simulink model "c00003M_harness"  (R2018a)
settings: Solver=FixedStepAuto  StartTime=0.0  StopTime=300  FixedStep=0.1  RelTol=1e-3
undefined symbols (not defined in the file): A1, hmax, PriorityTank, R1, R2, sigbuilder_block
(part 8 of 44)

== system c00003M_harness/M006/Tank1 ==
  CT1 : Inport
  F1 : Inport  Port=2
  E1 : Inport  Port=3
  MR1 : Inport  Port=4
  T1 : Inport  Port=5
  EB1 : Inport  Port=6
  LL2 : Inport  Port=7
  Control : Subsystem
  Logical Operator : Logic  AllPortsSameDT=off  OutDataTypeStr=boolean
  MasterTankControl : Subsystem
  Memory : Memory
  Memory1 : Memory
  TankModel : Subsystem
  LL1 : Outport
  wires:
  TankModel/1(LiquidLevel) -> Memory/1, LL1/1
  Control/1(LiquidIn) -> Logical Operator/1
  Control/2(LiquidOut) -> TankModel/2(LiquidOut)
  Memory/1 -> Control/7(LiquidLevel), MasterTankControl/1(LiquidTank1)
  MR1/1 -> Control/3(ManualReference)
  CT1/1 -> Control/2(StartMaintenance), Control/1(ControlType)
  F1/1 -> Control/4(Fill)
  E1/1 -> Control/5(Empty)
  Memory1/1 -> MasterTankControl/2(LiquidTank2)
  EB1/1 -> Control/6(EmergencyButton)
  MasterTankControl/1(AllowTheTankFilling) -> Logical Operator/2
  Logical Operator/1 -> TankModel/1(LiquidIn)
  LL2/1 -> Memory1/1

== system c00003M_harness/M006/Tank2 ==
  CT2 : Inport
  F2 : Inport  Port=2
  E2 : Inport  Port=3
  MR2 : Inport  Port=4
  T2 : Inport  Port=5
  EB2 : Inport  Port=6
  LL1 : Inport  Port=7
  Control : Subsystem
  Logical Operator : Logic  AllPortsSameDT=off  OutDataTypeStr=boolean
  MasterTankControl : Subsystem
  Memory : Memory
  Memory1 : Memory
  TankModel : Subsystem
  LL2 : Outport
  wires:
  TankModel/1(LiquidLevel) -> Memory/1, LL2/1
  Control/1(LiquidIn) -> Logical Operator/1
  Control/2(LiquidOut) -> TankModel/2(LiquidOut)
  Memory/1 -> Control/6(LiquidLevel), MasterTankControl/2(LiquidTank2)
  MR2/1 -> Control/2(ManualReference)
  CT2/1 -> Control/1(ControlType)
  F2/1 -> Control/3(Fill)
  E2/1 -> Control/4(Empty)
  Memory1/1 -> MasterTankControl/1(LiquidTank1)
  EB2/1 -> Control/5(EmergencyButton)
  MasterTankControl/1(AllowTheTankFilling) -> Logical Operator/2
  Logical Operator/1 -> TankModel/1(LiquidIn)
  LL1/1 -> Memory1/1

== system c00003M_harness/M007/Tank1 ==
  CT1 : Inport
  F1 : Inport  Port=2
  E1 : Inport  Port=3
  MR1 : Inport  Port=4
  T1 : Inport  Port=5
  EB1 : Inport  Port=6
  LL2 : Inport  Port=7
  Control : Subsystem
  Logical Operator : Logic  AllPortsSameDT=off  OutDataTypeStr=boolean
  MasterTankControl : Subsystem
  Memory : Memory
  Memory1 : Memory
  TankModel : Subsystem
  LL1 : Outport
  wires:
  TankModel/1(LiquidLevel) -> Memory/1, LL1/1
  Control/1(LiquidIn) -> Logical Operator/1
  Control/2(LiquidOut) -> TankModel/2(LiquidOut)
  Memory/1 -> Control/7(LiquidLevel), MasterTankControl/1(LiquidTank1)
  MR1/1 -> Control/3(ManualReference)
  CT1/1 -> Control/2(StartMaintenance), Control/1(ControlType)
  F1/1 -> Control/4(Fill)
  E1/1 -> Control/5(Empty)
  Memory1/1 -> MasterTankControl/2(LiquidTank2)
  EB1/1 -> Control/6(EmergencyButton)
  MasterTankControl/1(AllowTheTankFilling) -> Logical Operator/2
  Logical Operator/1 -> TankModel/1(LiquidIn)
  LL2/1 -> Memory1/1

== system c00003M_harness/M007/Tank2 ==
  CT2 : Inport
  F2 : Inport  Port=2
  E2 : Inport  Port=3
  MR2 : Inport  Port=4
  T2 : Inport  Port=5
  EB2 : Inport  Port=6
  LL1 : Inport  Port=7
  Control : Subsystem
  Logical Operator : Logic  AllPortsSameDT=off  OutDataTypeStr=boolean
  MasterTankControl : Subsystem
  Memory : Memory
  Memory1 : Memory
  TankModel : Subsystem
  LL2 : Outport
  wires:
  TankModel/1(LiquidLevel) -> Memory/1, LL2/1
  Control/1(LiquidIn) -> Logical Operator/1
  Control/2(LiquidOut) -> TankModel/2(LiquidOut)
  Memory/1 -> Control/6(LiquidLevel), MasterTankControl/2(LiquidTank2)
  MR2/1 -> Control/2(ManualReference)
  CT2/1 -> Control/1(ControlType)
  F2/1 -> Control/3(Fill)
  E2/1 -> Control/4(Empty)
  Memory1/1 -> MasterTankControl/1(LiquidTank1)
  EB2/1 -> Control/5(EmergencyButton)
  MasterTankControl/1(AllowTheTankFilling) -> Logical Operator/2
  Logical Operator/1 -> TankModel/1(LiquidIn)
  LL1/1 -> Memory1/1

== system c00003M_harness/M008/Tank1 ==
  CT1 : Inport
  F1 : Inport  Port=2
  E1 : Inport  Port=3
  MR1 : Inport  Port=4
  T1 : Inport  Port=5
  EB1 : Inport  Port=6
  LL2 : Inport  Port=7
  Control : Subsystem
  Logical Operator : Logic  AllPortsSameDT=off  OutDataTypeStr=boolean
  MasterTankControl : Subsystem
  Memory : Memory
  Memory1 : Memory
  TankModel : Subsystem
  LL1 : Outport
  wires:
  TankModel/1(LiquidLevel) -> Memory/1, LL1/1
  Control/1(LiquidIn) -> Logical Operator/1
  Control/2(LiquidOut) -> TankModel/2(LiquidOut)
  Memory/1 -> Control/7(LiquidLevel), MasterTankControl/1(LiquidTank1)
  MR1/1 -> Control/3(ManualReference)
  CT1/1 -> Control/2(StartMaintenance), Control/1(ControlType)
  F1/1 -> Control/4(Fill)
  E1/1 -> Control/5(Empty)
  Memory1/1 -> MasterTankControl/2(LiquidTank2)
  EB1/1 -> Control/6(EmergencyButton)
  MasterTankControl/1(AllowTheTankFilling) -> Logical Operator/2
  Logical Operator/1 -> TankModel/1(LiquidIn)
  LL2/1 -> Memory1/1

== system c00003M_harness/M008/Tank2 ==
  CT2 : Inport
  F2 : Inport  Port=2
  E2 : Inport  Port=3
  MR2 : Inport  Port=4
  T2 : Inport  Port=5
  EB2 : Inport  Port=6
  LL1 : Inport  Port=7
  Control : Subsystem
  Logical Operator : Logic  AllPortsSameDT=off  OutDataTypeStr=boolean
  MasterTankControl : Subsystem
  Memory : Memory
  Memory1 : Memory
  TankModel : Subsystem
  LL2 : Outport
  wires:
  TankModel/1(LiquidLevel) -> Memory/1, LL2/1
  Control/1(LiquidIn) -> Logical Operator/1
  Control/2(LiquidOut) -> TankModel/2(LiquidOut)
  Memory/1 -> Control/6(LiquidLevel), MasterTankControl/2(LiquidTank2)
  MR2/1 -> Control/2(ManualReference)
  CT2/1 -> Control/1(ControlType)
  F2/1 -> Control/3(Fill)
  E2/1 -> Control/4(Empty)
  Memory1/1 -> MasterTankControl/1(LiquidTank1)
  EB2/1 -> Control/5(EmergencyButton)
  MasterTankControl/1(AllowTheTankFilling) -> Logical Operator/2
  Logical Operator/1 -> TankModel/1(LiquidIn)
  LL1/1 -> Memory1/1

== system c00003M_harness/M009/Tank1 ==
  CT1 : Inport
  F1 : Inport  Port=2
  E1 : Inport  Port=3
  MR1 : Inport  Port=4
  T1 : Inport  Port=5
  EB1 : Inport  Port=6
  LL2 : Inport  Port=7
  Control : Subsystem
  Logical Operator : Logic  AllPortsSameDT=off  OutDataTypeStr=boolean
  MasterTankControl : Subsystem
  Memory : Memory
  Memory1 : Memory
  TankModel : Subsystem
  LL1 : Outport
  wires:
  TankModel/1(LiquidLevel) -> Memory/1, LL1/1
  Control/1(LiquidIn) -> Logical Operator/1
  Control/2(LiquidOut) -> TankModel/2(LiquidOut)
  Memory/1 -> Control/7(LiquidLevel), MasterTankControl/1(LiquidTank1)
  MR1/1 -> Control/3(ManualReference)
  CT1/1 -> Control/2(StartMaintenance), Control/1(ControlType)
  F1/1 -> Control/4(Fill)
  E1/1 -> Control/5(Empty)
  Memory1/1 -> MasterTankControl/2(LiquidTank2)
  EB1/1 -> Control/6(EmergencyButton)
  MasterTankControl/1(AllowTheTankFilling) -> Logical Operator/2
  Logical Operator/1 -> TankModel/1(LiquidIn)
  LL2/1 -> Memory1/1

== system c00003M_harness/M009/Tank2 ==
  CT2 : Inport
  F2 : Inport  Port=2
  E2 : Inport  Port=3
  MR2 : Inport  Port=4
  T2 : Inport  Port=5
  EB2 : Inport  Port=6
  LL1 : Inport  Port=7
  Control : Subsystem
  Logical Operator : Logic  AllPortsSameDT=off  OutDataTypeStr=boolean
  MasterTankControl : Subsystem
  Memory : Memory
  Memory1 : Memory
  TankModel : Subsystem
  LL2 : Outport
  wires:
  TankModel/1(LiquidLevel) -> Memory/1, LL2/1
  Control/1(LiquidIn) -> Logical Operator/1
  Control/2(LiquidOut) -> TankModel/2(LiquidOut)
  Memory/1 -> Control/6(LiquidLevel), MasterTankControl/2(LiquidTank2)
  MR2/1 -> Control/2(ManualReference)
  CT2/1 -> Control/1(ControlType)
  F2/1 -> Control/3(Fill)
  E2/1 -> Control/4(Empty)
  Memory1/1 -> MasterTankControl/1(LiquidTank1)
  EB2/1 -> Control/5(EmergencyButton)
  MasterTankControl/1(AllowTheTankFilling) -> Logical Operator/2
  Logical Operator/1 -> TankModel/1(LiquidIn)
  LL1/1 -> Memory1/1

== system c00003M_harness/M010/Tank1 ==
  CT1 : Inport
  F1 : Inport  Port=2
  E1 : Inport  Port=3
  MR1 : Inport  Port=4
  T1 : Inport  Port=5
  EB1 : Inport  Port=6
  LL2 : Inport  Port=7
  Control : Subsystem
  Logical Operator : Logic  AllPortsSameDT=off  OutDataTypeStr=boolean
  MasterTankControl : Subsystem
  Memory : Memory
  Memory1 : Memory
  TankModel : Subsystem
  LL1 : Outport
  wires:
  TankModel/1(LiquidLevel) -> Memory/1, LL1/1
  Control/1(LiquidIn) -> Logical Operator/1
  Control/2(LiquidOut) -> TankModel/2(LiquidOut)
  Memory/1 -> Control/7(LiquidLevel), MasterTankControl/1(LiquidTank1)
  MR1/1 -> Control/3(ManualReference)
  CT1/1 -> Control/2(StartMaintenance), Control/1(ControlType)
  F1/1 -> Control/4(Fill)
  E1/1 -> Control/5(Empty)
  Memory1/1 -> MasterTankControl/2(LiquidTank2)
  EB1/1 -> Control/6(EmergencyButton)
  MasterTankControl/1(AllowTheTankFilling) -> Logical Operator/2
  Logical Operator/1 -> TankModel/1(LiquidIn)
  LL2/1 -> Memory1/1

== system c00003M_harness/M010/Tank2 ==
  CT2 : Inport
  F2 : Inport  Port=2
  E2 : Inport  Port=3
  MR2 : Inport  Port=4
  T2 : Inport  Port=5
  EB2 : Inport  Port=6
  LL1 : Inport  Port=7
  Control : Subsystem
  Logical Operator : Logic  AllPortsSameDT=off  OutDataTypeStr=boolean
  MasterTankControl : Subsystem
  Memory : Memory
  Memory1 : Memory
  TankModel : Subsystem
  LL2 : Outport
  wires:
  TankModel/1(LiquidLevel) -> Memory/1, LL2/1
  Control/1(LiquidIn) -> Logical Operator/1
  Control/2(LiquidOut) -> TankModel/2(LiquidOut)
  Memory/1 -> Control/6(LiquidLevel), MasterTankControl/2(LiquidTank2)
  MR2/1 -> Control/2(ManualReference)
  CT2/1 -> Control/1(ControlType)
  F2/1 -> Control/3(Fill)
  E2/1 -> Control/4(Empty)
  Memory1/1 -> MasterTankControl/1(LiquidTank1)
  EB2/1 -> Control/5(EmergencyButton)
  MasterTankControl/1(AllowTheTankFilling) -> Logical Operator/2
  Logical Operator/1 -> TankModel/1(LiquidIn)
  LL1/1 -> Memory1/1

== system c00003M_harness/M011/Tank1 ==
  CT1 : Inport
  F1 : Inport  Port=2
  E1 : Inport  Port=3
  MR1 : Inport  Port=4
  T1 : Inport  Port=5
  EB1 : Inport  Port=6
  LL2 : Inport  Port=7
  Control : Subsystem
  Logical Operator : Logic  AllPortsSameDT=off  OutDataTypeStr=boolean
  MasterTankControl : Subsystem
  Memory : Memory
  Memory1 : Memory
  TankModel : Subsystem
  LL1 : Outport
  wires:
  TankModel/1(LiquidLevel) -> Memory/1, LL1/1
  Control/1(LiquidIn) -> Logical Operator/1
  Control/2(LiquidOut) -> TankModel/2(LiquidOut)
  Memory/1 -> Control/7(LiquidLevel), MasterTankControl/1(LiquidTank1)
  MR1/1 -> Control/3(ManualReference)
  CT1/1 -> Control/2(StartMaintenance), Control/1(ControlType)
  F1/1 -> Control/4(Fill)
  E1/1 -> Control/5(Empty)
  Memory1/1 -> MasterTankControl/2(LiquidTank2)
  EB1/1 -> Control/6(EmergencyButton)
  MasterTankControl/1(AllowTheTankFilling) -> Logical Operator/2
  Logical Operator/1 -> TankModel/1(LiquidIn)
  LL2/1 -> Memory1/1

== system c00003M_harness/M011/Tank2 ==
  CT2 : Inport
  F2 : Inport  Port=2
  E2 : Inport  Port=3
  MR2 : Inport  Port=4
  T2 : Inport  Port=5
  EB2 : Inport  Port=6
  LL1 : Inport  Port=7
  Control : Subsystem
  Logical Operator : Logic  AllPortsSameDT=off  OutDataTypeStr=boolean
  MasterTankControl : Subsystem
  Memory : Memory
  Memory1 : Memory
  TankModel : Subsystem
  LL2 : Outport
  wires:
  TankModel/1(LiquidLevel) -> Memory/1, LL2/1
  Control/1(LiquidIn) -> Logical Operator/1
  Control/2(LiquidOut) -> TankModel/2(LiquidOut)
  Memory/1 -> Control/6(LiquidLevel), MasterTankControl/2(LiquidTank2)
  MR2/1 -> Control/2(ManualReference)
  CT2/1 -> Control/1(ControlType)
  F2/1 -> Control/3(Fill)
  E2/1 -> Control/4(Empty)
  Memory1/1 -> MasterTankControl/1(LiquidTank1)
  EB2/1 -> Control/5(EmergencyButton)
  MasterTankControl/1(AllowTheTankFilling) -> Logical Operator/2
  Logical Operator/1 -> TankModel/1(LiquidIn)
  LL1/1 -> Memory1/1

== system c00003M_harness/M012/Tank1 ==
  CT1 : Inport
  F1 : Inport  Port=2
  E1 : Inport  Port=3
  MR1 : Inport  Port=4
  T1 : Inport  Port=5
  EB1 : Inport  Port=6
  LL2 : Inport  Port=7
  Control : Subsystem
  Logical Operator : Logic  AllPortsSameDT=off  OutDataTypeStr=boolean
  MasterTankControl : Subsystem
  Memory : Memory
  Memory1 : Memory
  TankModel : Subsystem
  LL1 : Outport
  wires:
  TankModel/1(LiquidLevel) -> Memory/1, LL1/1
  Control/1(LiquidIn) -> Logical Operator/1
  Control/2(LiquidOut) -> TankModel/2(LiquidOut)
  Memory/1 -> Control/7(LiquidLevel), MasterTankControl/1(LiquidTank1)
  MR1/1 -> Control/3(ManualReference)
  CT1/1 -> Control/2(StartMaintenance), Control/1(ControlType)
  F1/1 -> Control/4(Fill)
  E1/1 -> Control/5(Empty)
  Memory1/1 -> MasterTankControl/2(LiquidTank2)
  EB1/1 -> Control/6(EmergencyButton)
  MasterTankControl/1(AllowTheTankFilling) -> Logical Operator/2
  Logical Operator/1 -> TankModel/1(LiquidIn)
  LL2/1 -> Memory1/1

== system c00003M_harness/M012/Tank2 ==
  CT2 : Inport
  F2 : Inport  Port=2
  E2 : Inport  Port=3
  MR2 : Inport  Port=4
  T2 : Inport  Port=5
  EB2 : Inport  Port=6
  LL1 : Inport  Port=7
  Control : Subsystem
  Logical Operator : Logic  AllPortsSameDT=off  OutDataTypeStr=boolean
  MasterTankControl : Subsystem
  Memory : Memory
  Memory1 : Memory
  TankModel : Subsystem
  LL2 : Outport
  wires:
  TankModel/1(LiquidLevel) -> Memory/1, LL2/1
  Control/1(LiquidIn) -> Logical Operator/1
  Control/2(LiquidOut) -> TankModel/2(LiquidOut)
  Memory/1 -> Control/6(LiquidLevel), MasterTankControl/2(LiquidTank2)
  MR2/1 -> Control/2(ManualReference)
  CT2/1 -> Control/1(ControlType)
  F2/1 -> Control/3(Fill)
  E2/1 -> Control/4(Empty)
  Memory1/1 -> MasterTankControl/1(LiquidTank1)
  EB2/1 -> Control/5(EmergencyButton)
  MasterTankControl/1(AllowTheTankFilling) -> Logical Operator/2
  Logical Operator/1 -> TankModel/1(LiquidIn)
  LL1/1 -> Memory1/1

== system c00003M_harness/M013/Tank1 ==
  CT1 : Inport
  F1 : Inport  Port=2
  E1 : Inport  Port=3
  MR1 : Inport  Port=4
  T1 : Inport  Port=5
  EB1 : Inport  Port=6
  LL2 : Inport  Port=7
  Control : Subsystem
  Logical Operator : Logic  AllPortsSameDT=off  OutDataTypeStr=boolean
  MasterTankControl : Subsystem
  Memory : Memory
  Memory1 : Memory
  TankModel : Subsystem
  LL1 : Outport
  wires:
  TankModel/1(LiquidLevel) -> Memory/1, LL1/1
  Control/1(LiquidIn) -> Logical Operator/1
  Control/2(LiquidOut) -> TankModel/2(LiquidOut)
  Memory/1 -> Control/7(LiquidLevel), MasterTankControl/1(LiquidTank1)
  MR1/1 -> Control/3(ManualReference)
  CT1/1 -> Control/2(StartMaintenance), Control/1(ControlType)
  F1/1 -> Control/4(Fill)
  E1/1 -> Control/5(Empty)
  Memory1/1 -> MasterTankControl/2(LiquidTank2)
  EB1/1 -> Control/6(EmergencyButton)
  MasterTankControl/1(AllowTheTankFilling) -> Logical Operator/2
  Logical Operator/1 -> TankModel/1(LiquidIn)
  LL2/1 -> Memory1/1

== system c00003M_harness/M013/Tank2 ==
  CT2 : Inport
  F2 : Inport  Port=2
  E2 : Inport  Port=3
  MR2 : Inport  Port=4
  T2 : Inport  Port=5
  EB2 : Inport  Port=6
  LL1 : Inport  Port=7
  Control : Subsystem
  Logical Operator : Logic  AllPortsSameDT=off  OutDataTypeStr=boolean
  MasterTankControl : Subsystem
  Memory : Memory
  Memory1 : Memory
  TankModel : Subsystem
  LL2 : Outport
  wires:
  TankModel/1(LiquidLevel) -> Memory/1, LL2/1
  Control/1(LiquidIn) -> Logical Operator/1
  Control/2(LiquidOut) -> TankModel/2(LiquidOut)
  Memory/1 -> Control/6(LiquidLevel), MasterTankControl/2(LiquidTank2)
  MR2/1 -> Control/2(ManualReference)
  CT2/1 -> Control/1(ControlType)
  F2/1 -> Control/3(Fill)
  E2/1 -> Control/4(Empty)
  Memory1/1 -> MasterTankControl/1(LiquidTank1)
  EB2/1 -> Control/5(EmergencyButton)
  MasterTankControl/1(AllowTheTankFilling) -> Logical Operator/2
  Logical Operator/1 -> TankModel/1(LiquidIn)
  LL1/1 -> Memory1/1

== system c00003M_harness/M014/Tank1 ==
  CT1 : Inport
  F1 : Inport  Port=2
  E1 : Inport  Port=3
  MR1 : Inport  Port=4
  T1 : Inport  Port=5
  EB1 : Inport  Port=6
  LL2 : Inport  Port=7
  Control : Subsystem
  Logical Operator : Logic  AllPortsSameDT=off  OutDataTypeStr=boolean
  MasterTankControl : Subsystem
  Memory : Memory
  Memory1 : Memory
  TankModel : Subsystem
  LL1 : Outport
  wires:
  TankModel/1(LiquidLevel) -> Memory/1, LL1/1
  Control/1(LiquidIn) -> Logical Operator/1
  Control/2(LiquidOut) -> TankModel/2(LiquidOut)
  Memory/1 -> Control/7(LiquidLevel), MasterTankControl/1(LiquidTank1)
  MR1/1 -> Control/3(ManualReference)
  CT1/1 -> Control/2(StartMaintenance), Control/1(ControlType)
  F1/1 -> Control/4(Fill)
  E1/1 -> Control/5(Empty)
  Memory1/1 -> MasterTankControl/2(LiquidTank2)
  EB1/1 -> Control/6(EmergencyButton)
  MasterTankControl/1(AllowTheTankFilling) -> Logical Operator/2
  Logical Operator/1 -> TankModel/1(LiquidIn)
  LL2/1 -> Memory1/1

== system c00003M_harness/M014/Tank2 ==
  CT2 : Inport
  F2 : Inport  Port=2
  E2 : Inport  Port=3
  MR2 : Inport  Port=4
  T2 : Inport  Port=5
  EB2 : Inport  Port=6
  LL1 : Inport  Port=7
  Control : Subsystem
  Logical Operator : Logic  AllPortsSameDT=off  OutDataTypeStr=boolean
  MasterTankControl : Subsystem
  Memory : Memory
  Memory1 : Memory
  TankModel : Subsystem
  LL2 : Outport
  wires:
  TankModel/1(LiquidLevel) -> Memory/1, LL2/1
  Control/1(LiquidIn) -> Logical Operator/1
  Control/2(LiquidOut) -> TankModel/2(LiquidOut)
  Memory/1 -> Control/6(LiquidLevel), MasterTankControl/2(LiquidTank2)
  MR2/1 -> Control/2(ManualReference)
  CT2/1 -> Control/1(ControlType)
  F2/1 -> Control/3(Fill)
  E2/1 -> Control/4(Empty)
  Memory1/1 -> MasterTankControl/1(LiquidTank1)
  EB2/1 -> Control/5(EmergencyButton)
  MasterTankControl/1(AllowTheTankFilling) -> Logical Operator/2
  Logical Operator/1 -> TankModel/1(LiquidIn)
  LL1/1 -> Memory1/1

== system c00003M_harness/M015/Tank1 ==
  CT1 : Inport
  F1 : Inport  Port=2
  E1 : Inport  Port=3
  MR1 : Inport  Port=4
  T1 : Inport  Port=5
  EB1 : Inport  Port=6
  LL2 : Inport  Port=7
  Control : Subsystem
  Logical Operator : Logic  AllPortsSameDT=off  OutDataTypeStr=boolean
  MasterTankControl : Subsystem
  Memory : Memory
  Memory1 : Memory
  TankModel : Subsystem
  LL1 : Outport
  wires:
  TankModel/1(LiquidLevel) -> Memory/1, LL1/1
  Control/1(LiquidIn) -> Logical Operator/1
  Control/2(LiquidOut) -> TankModel/2(LiquidOut)
  Memory/1 -> Control/7(LiquidLevel), MasterTankControl/1(LiquidTank1)
  MR1/1 -> Control/3(ManualReference)
  CT1/1 -> Control/2(StartMaintenance), Control/1(ControlType)
  F1/1 -> Control/4(Fill)
  E1/1 -> Control/5(Empty)
  Memory1/1 -> MasterTankControl/2(LiquidTank2)
  EB1/1 -> Control/6(EmergencyButton)
  MasterTankControl/1(AllowTheTankFilling) -> Logical Operator/2
  Logical Operator/1 -> TankModel/1(LiquidIn)
  LL2/1 -> Memory1/1

== system c00003M_harness/M015/Tank2 ==
  CT2 : Inport
  F2 : Inport  Port=2
  E2 : Inport  Port=3
  MR2 : Inport  Port=4
  T2 : Inport  Port=5
  EB2 : Inport  Port=6
  LL1 : Inport  Port=7
  Control : Subsystem
  Logical Operator : Logic  AllPortsSameDT=off  OutDataTypeStr=boolean
  MasterTankControl : Subsystem
  Memory : Memory
  Memory1 : Memory
  TankModel : Subsystem
  LL2 : Outport
  wires:
  TankModel/1(LiquidLevel) -> Memory/1, LL2/1
  Control/1(LiquidIn) -> Logical Operator/1
  Control/2(LiquidOut) -> TankModel/2(LiquidOut)
  Memory/1 -> Control/6(LiquidLevel), MasterTankControl/2(LiquidTank2)
  MR2/1 -> Control/2(ManualReference)
  CT2/1 -> Control/1(ControlType)
  F2/1 -> Control/3(Fill)
  E2/1 -> Control/4(Empty)
  Memory1/1 -> MasterTankControl/1(LiquidTank1)
  EB2/1 -> Control/5(EmergencyButton)
  MasterTankControl/1(AllowTheTankFilling) -> Logical Operator/2
  Logical Operator/1 -> TankModel/1(LiquidIn)
  LL1/1 -> Memory1/1

== system c00003M_harness/M016/Tank1 ==
  CT1 : Inport
  F1 : Inport  Port=2
  E1 : Inport  Port=3
  MR1 : Inport  Port=4
  T1 : Inport  Port=5
  EB1 : Inport  Port=6
  LL2 : Inport  Port=7
  Control : Subsystem
  Logical Operator : Logic  AllPortsSameDT=off  OutDataTypeStr=boolean
  MasterTankControl : Subsystem
  Memory : Memory
  Memory1 : Memory
  TankModel : Subsystem
  LL1 : Outport
  wires:
  TankModel/1(LiquidLevel) -> Memory/1, LL1/1
  Control/1(LiquidIn) -> Logical Operator/1
  Control/2(LiquidOut) -> TankModel/2(LiquidOut)
  Memory/1 -> Control/7(LiquidLevel), MasterTankControl/1(LiquidTank1)
  MR1/1 -> Control/3(ManualReference)
  CT1/1 -> Control/2(StartMaintenance), Control/1(ControlType)
  F1/1 -> Control/4(Fill)
  E1/1 -> Control/5(Empty)
  Memory1/1 -> MasterTankControl/2(LiquidTank2)
  EB1/1 -> Control/6(EmergencyButton)
  MasterTankControl/1(AllowTheTankFilling) -> Logical Operator/2
  Logical Operator/1 -> TankModel/1(LiquidIn)
  LL2/1 -> Memory1/1

== system c00003M_harness/M016/Tank2 ==
  CT2 : Inport
  F2 : Inport  Port=2
  E2 : Inport  Port=3
  MR2 : Inport  Port=4
  T2 : Inport  Port=5
  EB2 : Inport  Port=6
  LL1 : Inport  Port=7
  Control : Subsystem
  Logical Operator : Logic  AllPortsSameDT=off  OutDataTypeStr=boolean
  MasterTankControl : Subsystem
  Memory : Memory
  Memory1 : Memory
  TankModel : Subsystem
  LL2 : Outport
  wires:
  TankModel/1(LiquidLevel) -> Memory/1, LL2/1
  Control/1(LiquidIn) -> Logical Operator/1
  Control/2(LiquidOut) -> TankModel/2(LiquidOut)
  Memory/1 -> Control/6(LiquidLevel), MasterTankControl/2(LiquidTank2)
  MR2/1 -> Control/2(ManualReference)
  CT2/1 -> Control/1(ControlType)
  F2/1 -> Control/3(Fill)
  E2/1 -> Control/4(Empty)
  Memory1/1 -> MasterTankControl/1(LiquidTank1)
  EB2/1 -> Control/5(EmergencyButton)
  MasterTankControl/1(AllowTheTankFilling) -> Logical Operator/2
  Logical Operator/1 -> TankModel/1(LiquidIn)
  LL1/1 -> Memory1/1

== system c00003M_harness/M017/Tank1 ==
  CT1 : Inport
  F1 : Inport  Port=2
  E1 : Inport  Port=3
  MR1 : Inport  Port=4
  T1 : Inport  Port=5
  EB1 : Inport  Port=6
  LL2 : Inport  Port=7
  Control : Subsystem
  Logical Operator : Logic  AllPortsSameDT=off  OutDataTypeStr=boolean
  MasterTankControl : Subsystem
  Memory : Memory
  Memory1 : Memory
  TankModel : Subsystem
  LL1 : Outport
  wires:
  TankModel/1(LiquidLevel) -> Memory/1, LL1/1
  Control/1(LiquidIn) -> Logical Operator/1
  Control/2(LiquidOut) -> TankModel/2(LiquidOut)
  Memory/1 -> Control/7(LiquidLevel), MasterTankControl/1(LiquidTank1)
  MR1/1 -> Control/3(ManualReference)
  CT1/1 -> Control/2(StartMaintenance), Control/1(ControlType)
  F1/1 -> Control/4(Fill)
  E1/1 -> Control/5(Empty)
  Memory1/1 -> MasterTankControl/2(LiquidTank2)
  EB1/1 -> Control/6(EmergencyButton)
  MasterTankControl/1(AllowTheTankFilling) -> Logical Operator/2
  Logical Operator/1 -> TankModel/1(LiquidIn)
  LL2/1 -> Memory1/1

== system c00003M_harness/M017/Tank2 ==
  CT2 : Inport
  F2 : Inport  Port=2
  E2 : Inport  Port=3
  MR2 : Inport  Port=4
  T2 : Inport  Port=5
  EB2 : Inport  Port=6
  LL1 : Inport  Port=7
  Control : Subsystem
  Logical Operator : Logic  AllPortsSameDT=off  OutDataTypeStr=boolean
  MasterTankControl : Subsystem
  Memory : Memory
  Memory1 : Memory
  TankModel : Subsystem
  LL2 : Outport
  wires:
  TankModel/1(LiquidLevel) -> Memory/1, LL2/1
  Control/1(LiquidIn) -> Logical Operator/1
  Control/2(LiquidOut) -> TankModel/2(LiquidOut)
  Memory/1 -> Control/6(LiquidLevel), MasterTankControl/2(LiquidTank2)
  MR2/1 -> Control/2(ManualReference)
  CT2/1 -> Control/1(ControlType)
  F2/1 -> Control/3(Fill)
  E2/1 -> Control/4(Empty)
  Memory1/1 -> MasterTankControl/1(LiquidTank1)
  EB2/1 -> Control/5(EmergencyButton)
  MasterTankControl/1(AllowTheTankFilling) -> Logical Operator/2
  Logical Operator/1 -> TankModel/1(LiquidIn)
  LL1/1 -> Memory1/1

== system c00003M_harness/M018/Tank1 ==
  CT1 : Inport
  F1 : Inport  Port=2
  E1 : Inport  Port=3
  MR1 : Inport  Port=4
  T1 : Inport  Port=5
  EB1 : Inport  Port=6
  LL2 : Inport  Port=7
  Control : Subsystem
  Logical Operator : Logic  AllPortsSameDT=off  OutDataTypeStr=boolean
  MasterTankControl : Subsystem
  Memory : Memory
  Memory1 : Memory
  TankModel : Subsystem
  LL1 : Outport
  wires:
  TankModel/1(LiquidLevel) -> Memory/1, LL1/1
  Control/1(LiquidIn) -> Logical Operator/1
  Control/2(LiquidOut) -> TankModel/2(LiquidOut)
  Memory/1 -> Control/7(LiquidLevel), MasterTankControl/1(LiquidTank1)
  MR1/1 -> Control/3(ManualReference)
  CT1/1 -> Control/2(StartMaintenance), Control/1(ControlType)
  F1/1 -> Control/4(Fill)
  E1/1 -> Control/5(Empty)
  Memory1/1 -> MasterTankControl/2(LiquidTank2)
  EB1/1 -> Control/6(EmergencyButton)
  MasterTankControl/1(AllowTheTankFilling) -> Logical Operator/2
  Logical Operator/1 -> TankModel/1(LiquidIn)
  LL2/1 -> Memory1/1

== system c00003M_harness/M018/Tank2 ==
  CT2 : Inport
  F2 : Inport  Port=2
  E2 : Inport  Port=3
  MR2 : Inport  Port=4
  T2 : Inport  Port=5
  EB2 : Inport  Port=6
  LL1 : Inport  Port=7
  Control : Subsystem
  Logical Operator : Logic  AllPortsSameDT=off  OutDataTypeStr=boolean
  MasterTankControl : Subsystem
  Memory : Memory
  Memory1 : Memory
  TankModel : Subsystem
  LL2 : Outport
  wires:
  TankModel/1(LiquidLevel) -> Memory/1, LL2/1
  Control/1(LiquidIn) -> Logical Operator/1
  Control/2(LiquidOut) -> TankModel/2(LiquidOut)
  Memory/1 -> Control/6(LiquidLevel), MasterTankControl/2(LiquidTank2)
  MR2/1 -> Control/2(ManualReference)
  CT2/1 -> Control/1(ControlType)
  F2/1 -> Control/3(Fill)
  E2/1 -> Control/4(Empty)
  Memory1/1 -> MasterTankControl/1(LiquidTank1)
  EB2/1 -> Control/5(EmergencyButton)
  MasterTankControl/1(AllowTheTankFilling) -> Logical Operator/2
  Logical Operator/1 -> TankModel/1(LiquidIn)
  LL1/1 -> Memory1/1

== system c00003M_harness/M019/Tank1 ==
  CT1 : Inport
  F1 : Inport  Port=2
  E1 : Inport  Port=3
  MR1 : Inport  Port=4
  T1 : Inport  Port=5
  EB1 : Inport  Port=6
  LL2 : Inport  Port=7
  Control : Subsystem
  Logical Operator : Logic  AllPortsSameDT=off  OutDataTypeStr=boolean
  MasterTankControl : Subsystem
  Memory : Memory
  Memory1 : Memory
  TankModel : Subsystem
  LL1 : Outport
  wires:
  TankModel/1(LiquidLevel) -> Memory/1, LL1/1
  Control/1(LiquidIn) -> Logical Operator/1
  Control/2(LiquidOut) -> TankModel/2(LiquidOut)
  Memory/1 -> Control/7(LiquidLevel), MasterTankControl/1(LiquidTank1)
  MR1/1 -> Control/3(ManualReference)
  CT1/1 -> Control/2(StartMaintenance), Control/1(ControlType)
  F1/1 -> Control/4(Fill)
  E1/1 -> Control/5(Empty)
  Memory1/1 -> MasterTankControl/2(LiquidTank2)
  EB1/1 -> Control/6(EmergencyButton)
  MasterTankControl/1(AllowTheTankFilling) -> Logical Operator/2
  Logical Operator/1 -> TankModel/1(LiquidIn)
  LL2/1 -> Memory1/1

== system c00003M_harness/M019/Tank2 ==
  CT2 : Inport
  F2 : Inport  Port=2
  E2 : Inport  Port=3
  MR2 : Inport  Port=4
  T2 : Inport  Port=5
  EB2 : Inport  Port=6
  LL1 : Inport  Port=7
  Control : Subsystem
  Logical Operator : Logic  AllPortsSameDT=off  OutDataTypeStr=boolean
  MasterTankControl : Subsystem
  Memory : Memory
  Memory1 : Memory
  TankModel : Subsystem
  LL2 : Outport
  wires:
  TankModel/1(LiquidLevel) -> Memory/1, LL2/1
  Control/1(LiquidIn) -> Logical Operator/1
  Control/2(LiquidOut) -> TankModel/2(LiquidOut)
  Memory/1 -> Control/6(LiquidLevel), MasterTankControl/2(LiquidTank2)
  MR2/1 -> Control/2(ManualReference)
  CT2/1 -> Control/1(ControlType)
  F2/1 -> Control/3(Fill)
  E2/1 -> Control/4(Empty)
  Memory1/1 -> MasterTankControl/1(LiquidTank1)
  EB2/1 -> Control/5(EmergencyButton)
  MasterTankControl/1(AllowTheTankFilling) -> Logical Operator/2
  Logical Operator/1 -> TankModel/1(LiquidIn)
  LL1/1 -> Memory1/1

== system c00003M_harness/M020/Tank1 ==
  CT1 : Inport
  F1 : Inport  Port=2
  E1 : Inport  Port=3
  MR1 : Inport  Port=4
  T1 : Inport  Port=5
  EB1 : Inport  Port=6
  LL2 : Inport  Port=7
  Control : Subsystem
  Logical Operator : Logic  AllPortsSameDT=off  OutDataTypeStr=boolean
  MasterTankControl : Subsystem
  Memory : Memory
  Memory1 : Memory
  TankModel : Subsystem
  LL1 : Outport
  wires:
  TankModel/1(LiquidLevel) -> Memory/1, LL1/1
  Control/1(LiquidIn) -> Logical Operator/1
  Control/2(LiquidOut) -> TankModel/2(LiquidOut)
  Memory/1 -> Control/7(LiquidLevel), MasterTankControl/1(LiquidTank1)
  MR1/1 -> Control/3(ManualReference)
  CT1/1 -> Control/2(StartMaintenance), Control/1(ControlType)
  F1/1 -> Control/4(Fill)
  E1/1 -> Control/5(Empty)
  Memory1/1 -> MasterTankControl/2(LiquidTank2)
  EB1/1 -> Control/6(EmergencyButton)
  MasterTankControl/1(AllowTheTankFilling) -> Logical Operator/2
  Logical Operator/1 -> TankModel/1(LiquidIn)
  LL2/1 -> Memory1/1

== system c00003M_harness/M020/Tank2 ==
  CT2 : Inport
  F2 : Inport  Port=2
  E2 : Inport  Port=3
  MR2 : Inport  Port=4
  T2 : Inport  Port=5
  EB2 : Inport  Port=6
  LL1 : Inport  Port=7
  Control : Subsystem
  Logical Operator : Logic  AllPortsSameDT=off  OutDataTypeStr=boolean
  MasterTankControl : Subsystem
  Memory : Memory
  Memory1 : Memory
  TankModel : Subsystem
  LL2 : Outport
  wires:
  TankModel/1(LiquidLevel) -> Memory/1, LL2/1
  Control/1(LiquidIn) -> Logical Operator/1
  Control/2(LiquidOut) -> TankModel/2(LiquidOut)
  Memory/1 -> Control/6(LiquidLevel), MasterTankControl/2(LiquidTank2)
  MR2/1 -> Control/2(ManualReference)
  CT2/1 -> Control/1(ControlType)
  F2/1 -> Control/3(Fill)
  E2/1 -> Control/4(Empty)
  Memory1/1 -> MasterTankControl/1(LiquidTank1)
  EB2/1 -> Control/5(EmergencyButton)
  MasterTankControl/1(AllowTheTankFilling) -> Logical Operator/2
  Logical Operator/1 -> TankModel/1(LiquidIn)
  LL1/1 -> Memory1/1

== system c00003M_harness/M021/Tank1 ==
  CT1 : Inport
  F1 : Inport  Port=2
  E1 : Inport  Port=3
  MR1 : Inport  Port=4
  T1 : Inport  Port=5
  EB1 : Inport  Port=6
  LL2 : Inport  Port=7
  Control : Subsystem
  Logical Operator : Logic  AllPortsSameDT=off  OutDataTypeStr=boolean
  MasterTankControl : Subsystem
  Memory : Memory
  Memory1 : Memory
  TankModel : Subsystem
  LL1 : Outport
  wires:
  TankModel/1(LiquidLevel) -> Memory/1, LL1/1
  Control/1(LiquidIn) -> Logical Operator/1
  Control/2(LiquidOut) -> TankModel/2(LiquidOut)
  Memory/1 -> Control/7(LiquidLevel), MasterTankControl/1(LiquidTank1)
  MR1/1 -> Control/3(ManualReference)
  CT1/1 -> Control/2(StartMaintenance), Control/1(ControlType)
  F1/1 -> Control/4(Fill)
  E1/1 -> Control/5(Empty)
  Memory1/1 -> MasterTankControl/2(LiquidTank2)
  EB1/1 -> Control/6(EmergencyButton)
  MasterTankControl/1(AllowTheTankFilling) -> Logical Operator/2
  Logical Operator/1 -> TankModel/1(LiquidIn)
  LL2/1 -> Memory1/1

== system c00003M_harness/M021/Tank2 ==
  CT2 : Inport
  F2 : Inport  Port=2
  E2 : Inport  Port=3
  MR2 : Inport  Port=4
  T2 : Inport  Port=5
  EB2 : Inport  Port=6
  LL1 : Inport  Port=7
  Control : Subsystem
  Logical Operator : Logic  AllPortsSameDT=off  OutDataTypeStr=boolean
  MasterTankControl : Subsystem
  Memory : Memory
  Memory1 : Memory
  TankModel : Subsystem
  LL2 : Outport
  wires:
  TankModel/1(LiquidLevel) -> Memory/1, LL2/1
  Control/1(LiquidIn) -> Logical Operator/1
  Control/2(LiquidOut) -> TankModel/2(LiquidOut)
  Memory/1 -> Control/6(LiquidLevel), MasterTankControl/2(LiquidTank2)
  MR2/1 -> Control/2(ManualReference)
  CT2/1 -> Control/1(ControlType)
  F2/1 -> Control/3(Fill)
  E2/1 -> Control/4(Empty)
  Memory1/1 -> MasterTankControl/1(LiquidTank1)
  EB2/1 -> Control/5(EmergencyButton)
  MasterTankControl/1(AllowTheTankFilling) -> Logical Operator/2
  Logical Operator/1 -> TankModel/1(LiquidIn)
  LL1/1 -> Memory1/1

== system c00003M_harness/M022/Tank1 ==
  CT1 : Inport
  F1 : Inport  Port=2
  E1 : Inport  Port=3
  MR1 : Inport  Port=4
  T1 : Inport  Port=5
  EB1 : Inport  Port=6
  LL2 : Inport  Port=7
  Control : Subsystem
  Logical Operator : Logic  AllPortsSameDT=off  OutDataTypeStr=boolean
  MasterTankControl : Subsystem
  Memory : Memory
  Memory1 : Memory
  TankModel : Subsystem
  LL1 : Outport
  wires:
  TankModel/1(LiquidLevel) -> Memory/1, LL1/1
  Control/1(LiquidIn) -> Logical Operator/1
  Control/2(LiquidOut) -> TankModel/2(LiquidOut)
  Memory/1 -> Control/7(LiquidLevel), MasterTankControl/1(LiquidTank1)
  MR1/1 -> Control/3(ManualReference)
  CT1/1 -> Control/2(StartMaintenance), Control/1(ControlType)
  F1/1 -> Control/4(Fill)
  E1/1 -> Control/5(Empty)
  Memory1/1 -> MasterTankControl/2(LiquidTank2)
  EB1/1 -> Control/6(EmergencyButton)
  MasterTankControl/1(AllowTheTankFilling) -> Logical Operator/2
  Logical Operator/1 -> TankModel/1(LiquidIn)
  LL2/1 -> Memory1/1

== system c00003M_harness/M022/Tank2 ==
  CT2 : Inport
  F2 : Inport  Port=2
  E2 : Inport  Port=3
  MR2 : Inport  Port=4
  T2 : Inport  Port=5
  EB2 : Inport  Port=6
  LL1 : Inport  Port=7
  Control : Subsystem
  Logical Operator : Logic  AllPortsSameDT=off  OutDataTypeStr=boolean
  MasterTankControl : Subsystem
  Memory : Memory
  Memory1 : Memory
  TankModel : Subsystem
  LL2 : Outport
  wires:
  TankModel/1(LiquidLevel) -> Memory/1, LL2/1
  Control/1(LiquidIn) -> Logical Operator/1
  Control/2(LiquidOut) -> TankModel/2(LiquidOut)
  Memory/1 -> Control/6(LiquidLevel), MasterTankControl/2(LiquidTank2)
  MR2/1 -> Control/2(ManualReference)
  CT2/1 -> Control/1(ControlType)
  F2/1 -> Control/3(Fill)
  E2/1 -> Control/4(Empty)
  Memory1/1 -> MasterTankControl/1(LiquidTank1)
  EB2/1 -> Control/5(EmergencyButton)
  MasterTankControl/1(AllowTheTankFilling) -> Logical Operator/2
  Logical Operator/1 -> TankModel/1(LiquidIn)
  LL1/1 -> Memory1/1

== system c00003M_harness/M023/Tank1 ==
  CT1 : Inport
  F1 : Inport  Port=2
  E1 : Inport  Port=3
  MR1 : Inport  Port=4
  T1 : Inport  Port=5
  EB1 : Inport  Port=6
  LL2 : Inport  Port=7
  Control : Subsystem
  Logical Operator : Logic  AllPortsSameDT=off  OutDataTypeStr=boolean
  MasterTankControl : Subsystem
  Memory : Memory
  Memory1 : Memory
  TankModel : Subsystem
  LL1 : Outport
  wires:
  TankModel/1(LiquidLevel) -> Memory/1, LL1/1
  Control/1(LiquidIn) -> Logical Operator/1
  Control/2(LiquidOut) -> TankModel/2(LiquidOut)
  Memory/1 -> Control/7(LiquidLevel), MasterTankControl/1(LiquidTank1)
  MR1/1 -> Control/3(ManualReference)
  CT1/1 -> Control/2(StartMaintenance), Control/1(ControlType)
  F1/1 -> Control/4(Fill)
  E1/1 -> Control/5(Empty)
  Memory1/1 -> MasterTankControl/2(LiquidTank2)
  EB1/1 -> Control/6(EmergencyButton)
  MasterTankControl/1(AllowTheTankFilling) -> Logical Operator/2
  Logical Operator/1 -> TankModel/1(LiquidIn)
  LL2/1 -> Memory1/1

== system c00003M_harness/M023/Tank2 ==
  CT2 : Inport
  F2 : Inport  Port=2
  E2 : Inport  Port=3
  MR2 : Inport  Port=4
  T2 : Inport  Port=5
  EB2 : Inport  Port=6
  LL1 : Inport  Port=7
  Control : Subsystem
  Logical Operator : Logic  AllPortsSameDT=off  OutDataTypeStr=boolean
  MasterTankControl : Subsystem
  Memory : Memory
  Memory1 : Memory
  TankModel : Subsystem
  LL2 : Outport
  wires:
  TankModel/1(LiquidLevel) -> Memory/1, LL2/1
  Control/1(LiquidIn) -> Logical Operator/1
  Control/2(LiquidOut) -> TankModel/2(LiquidOut)
  Memory/1 -> Control/6(LiquidLevel), MasterTankControl/2(LiquidTank2)
  MR2/1 -> Control/2(ManualReference)
  CT2/1 -> Control/1(ControlType)
  F2/1 -> Control/3(Fill)
  E2/1 -> Control/4(Empty)
  Memory1/1 -> MasterTankControl/1(LiquidTank1)
  EB2/1 -> Control/5(EmergencyButton)
  MasterTankControl/1(AllowTheTankFilling) -> Logical Operator/2
  Logical Operator/1 -> TankModel/1(LiquidIn)
  LL1/1 -> Memory1/1

== system c00003M_harness/M024/Tank1 ==
  CT1 : Inport
  F1 : Inport  Port=2
  E1 : Inport  Port=3
  MR1 : Inport  Port=4
  T1 : Inport  Port=5
  EB1 : Inport  Port=6
  LL2 : Inport  Port=7
  Control : Subsystem
  Logical Operator : Logic  AllPortsSameDT=off  OutDataTypeStr=boolean
  MasterTankControl : Subsystem
  Memory : Memory
  Memory1 : Memory
  TankModel : Subsystem
  LL1 : Outport
  wires:
  TankModel/1(LiquidLevel) -> Memory/1, LL1/1
  Control/1(LiquidIn) -> Logical Operator/1
  Control/2(LiquidOut) -> TankModel/2(LiquidOut)
  Memory/1 -> Control/7(LiquidLevel), MasterTankControl/1(LiquidTank1)
  MR1/1 -> Control/3(ManualReference)
  CT1/1 -> Control/2(StartMaintenance), Control/1(ControlType)
  F1/1 -> Control/4(Fill)
  E1/1 -> Control/5(Empty)
  Memory1/1 -> MasterTankControl/2(LiquidTank2)
  EB1/1 -> Control/6(EmergencyButton)
  MasterTankControl/1(AllowTheTankFilling) -> Logical Operator/2
  Logical Operator/1 -> TankModel/1(LiquidIn)
  LL2/1 -> Memory1/1

== system c00003M_harness/M024/Tank2 ==
  CT2 : Inport
  F2 : Inport  Port=2
  E2 : Inport  Port=3
  MR2 : Inport  Port=4
  T2 : Inport  Port=5
  EB2 : Inport  Port=6
  LL1 : Inport  Port=7
  Control : Subsystem
  Logical Operator : Logic  AllPortsSameDT=off  OutDataTypeStr=boolean
  MasterTankControl : Subsystem
  Memory : Memory
  Memory1 : Memory
  TankModel : Subsystem
  LL2 : Outport
  wires:
  TankModel/1(LiquidLevel) -> Memory/1, LL2/1
  Control/1(LiquidIn) -> Logical Operator/1
  Control/2(LiquidOut) -> TankModel/2(LiquidOut)
  Memory/1 -> Control/6(LiquidLevel), MasterTankControl/2(LiquidTank2)
  MR2/1 -> Control/2(ManualReference)
  CT2/1 -> Control/1(ControlType)
  F2/1 -> Control/3(Fill)
  E2/1 -> Control/4(Empty)
  Memory1/1 -> MasterTankControl/1(LiquidTank1)
  EB2/1 -> Control/5(EmergencyButton)
  MasterTankControl/1(AllowTheTankFilling) -> Logical Operator/2
  Logical Operator/1 -> TankModel/1(LiquidIn)
  LL1/1 -> Memory1/1

== system c00003M_harness/M025/Tank1 ==
  CT1 : Inport
  F1 : Inport  Port=2
  E1 : Inport  Port=3
  MR1 : Inport  Port=4
  T1 : Inport  Port=5
  EB1 : Inport  Port=6
  LL2 : Inport  Port=7
  Control : Subsystem
  Logical Operator : Logic  AllPortsSameDT=off  OutDataTypeStr=boolean
  MasterTankControl : Subsystem
  Memory : Memory
  Memory1 : Memory
  TankModel : Subsystem
  LL1 : Outport
  wires:
  TankModel/1(LiquidLevel) -> Memory/1, LL1/1
  Control/1(LiquidIn) -> Logical Operator/1
  Control/2(LiquidOut) -> TankModel/2(LiquidOut)
  Memory/1 -> Control/7(LiquidLevel), MasterTankControl/1(LiquidTank1)
  MR1/1 -> Control/3(ManualReference)
  CT1/1 -> Control/2(StartMaintenance), Control/1(ControlType)
  F1/1 -> Control/4(Fill)
  E1/1 -> Control/5(Empty)
  Memory1/1 -> MasterTankControl/2(LiquidTank2)
  EB1/1 -> Control/6(EmergencyButton)
  MasterTankControl/1(AllowTheTankFilling) -> Logical Operator/2
  Logical Operator/1 -> TankModel/1(LiquidIn)
  LL2/1 -> Memory1/1

== system c00003M_harness/M025/Tank2 ==
  CT2 : Inport
  F2 : Inport  Port=2
  E2 : Inport  Port=3
  MR2 : Inport  Port=4
  T2 : Inport  Port=5
  EB2 : Inport  Port=6
  LL1 : Inport  Port=7
  Control : Subsystem
  Logical Operator : Logic  AllPortsSameDT=off  OutDataTypeStr=boolean
  MasterTankControl : Subsystem
  Memory : Memory
  Memory1 : Memory
  TankModel : Subsystem
  LL2 : Outport
  wires:
  TankModel/1(LiquidLevel) -> Memory/1, LL2/1
  Control/1(LiquidIn) -> Logical Operator/1
  Control/2(LiquidOut) -> TankModel/2(LiquidOut)
  Memory/1 -> Control/6(LiquidLevel), MasterTankControl/2(LiquidTank2)
  MR2/1 -> Control/2(ManualReference)
  CT2/1 -> Control/1(ControlType)
  F2/1 -> Control/3(Fill)
  E2/1 -> Control/4(Empty)
  Memory1/1 -> MasterTankControl/1(LiquidTank1)
  EB2/1 -> Control/5(EmergencyButton)
  MasterTankControl/1(AllowTheTankFilling) -> Logical Operator/2
  Logical Operator/1 -> TankModel/1(LiquidIn)
  LL1/1 -> Memory1/1

== system c00003M_harness/M026/Tank1 ==
  CT1 : Inport
  F1 : Inport  Port=2
  E1 : Inport  Port=3
  MR1 : Inport  Port=4
  T1 : Inport  Port=5
  EB1 : Inport  Port=6
  LL2 : Inport  Port=7
  Control : Subsystem
  Logical Operator : Logic  AllPortsSameDT=off  OutDataTypeStr=boolean
  MasterTankControl : Subsystem
  Memory : Memory
  Memory1 : Memory
  TankModel : Subsystem
  LL1 : Outport
  wires:
  TankModel/1(LiquidLevel) -> Memory/1, LL1/1
  Control/1(LiquidIn) -> Logical Operator/1
  Control/2(LiquidOut) -> TankModel/2(LiquidOut)
  Memory/1 -> Control/7(LiquidLevel), MasterTankControl/1(LiquidTank1)
  MR1/1 -> Control/3(ManualReference)
  CT1/1 -> Control/2(StartMaintenance), Control/1(ControlType)
  F1/1 -> Control/4(Fill)
  E1/1 -> Control/5(Empty)
  Memory1/1 -> MasterTankControl/2(LiquidTank2)
  EB1/1 -> Control/6(EmergencyButton)
  MasterTankControl/1(AllowTheTankFilling) -> Logical Operator/2
  Logical Operator/1 -> TankModel/1(LiquidIn)
  LL2/1 -> Memory1/1

== system c00003M_harness/M026/Tank2 ==
  CT2 : Inport
  F2 : Inport  Port=2
  E2 : Inport  Port=3
  MR2 : Inport  Port=4
  T2 : Inport  Port=5
  EB2 : Inport  Port=6
  LL1 : Inport  Port=7
  Control : Subsystem
  Logical Operator : Logic  AllPortsSameDT=off  OutDataTypeStr=boolean
  MasterTankControl : Subsystem
  Memory : Memory
  Memory1 : Memory
  TankModel : Subsystem
  LL2 : Outport
  wires:
  TankModel/1(LiquidLevel) -> Memory/1, LL2/1
  Control/1(LiquidIn) -> Logical Operator/1
  Control/2(LiquidOut) -> TankModel/2(LiquidOut)
  Memory/1 -> Control/6(LiquidLevel), MasterTankControl/2(LiquidTank2)
  MR2/1 -> Control/2(ManualReference)
  CT2/1 -> Control/1(ControlType)
  F2/1 -> Control/3(Fill)
  E2/1 -> Control/4(Empty)
  Memory1/1 -> MasterTankControl/1(LiquidTank1)
  EB2/1 -> Control/5(EmergencyButton)
  MasterTankControl/1(AllowTheTankFilling) -> Logical Operator/2
  Logical Operator/1 -> TankModel/1(LiquidIn)
  LL1/1 -> Memory1/1

== system c00003M_harness/M027/Tank1 ==
  CT1 : Inport
  F1 : Inport  Port=2
  E1 : Inport  Port=3
  MR1 : Inport  Port=4
  T1 : Inport  Port=5
  EB1 : Inport  Port=6
  LL2 : Inport  Port=7
  Control : Subsystem
  Logical Operator : Logic  AllPortsSameDT=off  OutDataTypeStr=boolean
  MasterTankControl : Subsystem
  Memory : Memory
  Memory1 : Memory
  TankModel : Subsystem
  LL1 : Outport
  wires:
  TankModel/1(LiquidLevel) -> Memory/1, LL1/1
  Control/1(LiquidIn) -> Logical Operator/1
  Control/2(LiquidOut) -> TankModel/2(LiquidOut)
  Memory/1 -> Control/7(LiquidLevel), MasterTankControl/1(LiquidTank1)
  MR1/1 -> Control/3(ManualReference)
  CT1/1 -> Control/2(StartMaintenance), Control/1(ControlType)
  F1/1 -> Control/4(Fill)
  E1/1 -> Control/5(Empty)
  Memory1/1 -> MasterTankControl/2(LiquidTank2)
  EB1/1 -> Control/6(EmergencyButton)
  MasterTankControl/1(AllowTheTankFilling) -> Logical Operator/2
  Logical Operator/1 -> TankModel/1(LiquidIn)
  LL2/1 -> Memory1/1

== system c00003M_harness/M027/Tank2 ==
  CT2 : Inport
  F2 : Inport  Port=2
  E2 : Inport  Port=3
  MR2 : Inport  Port=4
  T2 : Inport  Port=5
  EB2 : Inport  Port=6
  LL1 : Inport  Port=7
  Control : Subsystem
  Logical Operator : Logic  AllPortsSameDT=off  OutDataTypeStr=boolean
  MasterTankControl : Subsystem
  Memory : Memory
  Memory1 : Memory
  TankModel : Subsystem
  LL2 : Outport
  wires:
  TankModel/1(LiquidLevel) -> Memory/1, LL2/1
  Control/1(LiquidIn) -> Logical Operator/1
  Control/2(LiquidOut) -> TankModel/2(LiquidOut)
  Memory/1 -> Control/6(LiquidLevel), MasterTankControl/2(LiquidTank2)
  MR2/1 -> Control/2(ManualReference)
  CT2/1 -> Control/1(ControlType)
  F2/1 -> Control/3(Fill)
  E2/1 -> Control/4(Empty)
  Memory1/1 -> MasterTankControl/1(LiquidTank1)
  EB2/1 -> Control/5(EmergencyButton)
  MasterTankControl/1(AllowTheTankFilling) -> Logical Operator/2
  Logical Operator/1 -> TankModel/1(LiquidIn)
  LL1/1 -> Memory1/1

== system c00003M_harness/M028/Tank1 ==
  CT1 : Inport
  F1 : Inport  Port=2
  E1 : Inport  Port=3
  MR1 : Inport  Port=4
  T1 : Inport  Port=5
  EB1 : Inport  Port=6
  LL2 : Inport  Port=7
  Control : Subsystem
  Logical Operator : Logic  AllPortsSameDT=off  OutDataTypeStr=boolean
  MasterTankControl : Subsystem
  Memory : Memory
  Memory1 : Memory
  TankModel : Subsystem
  LL1 : Outport
  wires:
  TankModel/1(LiquidLevel) -> Memory/1, LL1/1
  Control/1(LiquidIn) -> Logical Operator/1
  Control/2(LiquidOut) -> TankModel/2(LiquidOut)
  Memory/1 -> Control/7(LiquidLevel), MasterTankControl/1(LiquidTank1)
  MR1/1 -> Control/3(ManualReference)
  CT1/1 -> Control/2(StartMaintenance), Control/1(ControlType)
  F1/1 -> Control/4(Fill)
  E1/1 -> Control/5(Empty)
  Memory1/1 -> MasterTankControl/2(LiquidTank2)
  EB1/1 -> Control/6(EmergencyButton)
  MasterTankControl/1(AllowTheTankFilling) -> Logical Operator/2
  Logical Operator/1 -> TankModel/1(LiquidIn)
  LL2/1 -> Memory1/1

== system c00003M_harness/M028/Tank2 ==
  CT2 : Inport
  F2 : Inport  Port=2
  E2 : Inport  Port=3
  MR2 : Inport  Port=4
  T2 : Inport  Port=5
  EB2 : Inport  Port=6
  LL1 : Inport  Port=7
  Control : Subsystem
  Logical Operator : Logic  AllPortsSameDT=off  OutDataTypeStr=boolean
  MasterTankControl : Subsystem
  Memory : Memory
  Memory1 : Memory
  TankModel : Subsystem
  LL2 : Outport
  wires:
  TankModel/1(LiquidLevel) -> Memory/1, LL2/1
  Control/1(LiquidIn) -> Logical Operator/1
  Control/2(LiquidOut) -> TankModel/2(LiquidOut)
  Memory/1 -> Control/6(LiquidLevel), MasterTankControl/2(LiquidTank2)
  MR2/1 -> Control/2(ManualReference)
  CT2/1 -> Control/1(ControlType)
  F2/1 -> Control/3(Fill)
  E2/1 -> Control/4(Empty)
  Memory1/1 -> MasterTankControl/1(LiquidTank1)
  EB2/1 -> Control/5(EmergencyButton)
  MasterTankControl/1(AllowTheTankFilling) -> Logical Operator/2
  Logical Operator/1 -> TankModel/1(LiquidIn)
  LL1/1 -> Memory1/1

== system c00003M_harness/M029/Tank1 ==
  CT1 : Inport
  F1 : Inport  Port=2
  E1 : Inport  Port=3
  MR1 : Inport  Port=4
  T1 : Inport  Port=5
  EB1 : Inport  Port=6
  LL2 : Inport  Port=7
  Control : Subsystem
  Logical Operator : Logic  AllPortsSameDT=off  OutDataTypeStr=boolean
  MasterTankControl : Subsystem
  Memory : Memory
  Memory1 : Memory
  TankModel : Subsystem
  LL1 : Outport
  wires:
  TankModel/1(LiquidLevel) -> Memory/1, LL1/1
  Control/1(LiquidIn) -> Logical Operator/1
  Control/2(LiquidOut) -> TankModel/2(LiquidOut)
  Memory/1 -> Control/7(LiquidLevel), MasterTankControl/1(LiquidTank1)
  MR1/1 -> Control/3(ManualReference)
  CT1/1 -> Control/2(StartMaintenance), Control/1(ControlType)
  F1/1 -> Control/4(Fill)
  E1/1 -> Control/5(Empty)
  Memory1/1 -> MasterTankControl/2(LiquidTank2)
  EB1/1 -> Control/6(EmergencyButton)
  MasterTankControl/1(AllowTheTankFilling) -> Logical Operator/2
  Logical Operator/1 -> TankModel/1(LiquidIn)
  LL2/1 -> Memory1/1

== system c00003M_harness/M029/Tank2 ==
  CT2 : Inport
  F2 : Inport  Port=2
  E2 : Inport  Port=3
  MR2 : Inport  Port=4
  T2 : Inport  Port=5
  EB2 : Inport  Port=6
  LL1 : Inport  Port=7
  Control : Subsystem
  Logical Operator : Logic  AllPortsSameDT=off  OutDataTypeStr=boolean
  MasterTankControl : Subsystem
  Memory : Memory
  Memory1 : Memory
  TankModel : Subsystem
  LL2 : Outport
  wires:
  TankModel/1(LiquidLevel) -> Memory/1, LL2/1
  Control/1(LiquidIn) -> Logical Operator/1
  Control/2(LiquidOut) -> TankModel/2(LiquidOut)
  Memory/1 -> Control/6(LiquidLevel), MasterTankControl/2(LiquidTank2)
  MR2/1 -> Control/2(ManualReference)
  CT2/1 -> Control/1(ControlType)
  F2/1 -> Control/3(Fill)
  E2/1 -> Control/4(Empty)
  Memory1/1 -> MasterTankControl/1(LiquidTank1)
  EB2/1 -> Control/5(EmergencyButton)
  MasterTankControl/1(AllowTheTankFilling) -> Logical Operator/2
  Logical Operator/1 -> TankModel/1(LiquidIn)
  LL1/1 -> Memory1/1

== system c00003M_harness/M030/Tank1 ==
  CT1 : Inport
  F1 : Inport  Port=2
  E1 : Inport  Port=3
  MR1 : Inport  Port=4
  T1 : Inport  Port=5
  EB1 : Inport  Port=6
  LL2 : Inport  Port=7
  Control : Subsystem
  Logical Operator : Logic  AllPortsSameDT=off  OutDataTypeStr=boolean
  MasterTankControl : Subsystem
  Memory : Memory
  Memory1 : Memory
  TankModel : Subsystem
  LL1 : Outport
  wires:
  TankModel/1(LiquidLevel) -> Memory/1, LL1/1
  Control/1(LiquidIn) -> Logical Operator/1
  Control/2(LiquidOut) -> TankModel/2(LiquidOut)
  Memory/1 -> Control/7(LiquidLevel), MasterTankControl/1(LiquidTank1)
  MR1/1 -> Control/3(ManualReference)
  CT1/1 -> Control/2(StartMaintenance), Control/1(ControlType)
  F1/1 -> Control/4(Fill)
  E1/1 -> Control/5(Empty)
  Memory1/1 -> MasterTankControl/2(LiquidTank2)
  EB1/1 -> Control/6(EmergencyButton)
  MasterTankControl/1(AllowTheTankFilling) -> Logical Operator/2
  Logical Operator/1 -> TankModel/1(LiquidIn)
  LL2/1 -> Memory1/1

== system c00003M_harness/M030/Tank2 ==
  CT2 : Inport
  F2 : Inport  Port=2
  E2 : Inport  Port=3
  MR2 : Inport  Port=4
  T2 : Inport  Port=5
  EB2 : Inport  Port=6
  LL1 : Inport  Port=7
  Control : Subsystem
  Logical Operator : Logic  AllPortsSameDT=off  OutDataTypeStr=boolean
  MasterTankControl : Subsystem
  Memory : Memory
  Memory1 : Memory
  TankModel : Subsystem
  LL2 : Outport
  wires:
  TankModel/1(LiquidLevel) -> Memory/1, LL2/1
  Control/1(LiquidIn) -> Logical Operator/1
  Control/2(LiquidOut) -> TankModel/2(LiquidOut)
  Memory/1 -> Control/6(LiquidLevel), MasterTankControl/2(LiquidTank2)
  MR2/1 -> Control/2(ManualReference)
  CT2/1 -> Control/1(ControlType)
  F2/1 -> Control/3(Fill)
  E2/1 -> Control/4(Empty)
  Memory1/1 -> MasterTankControl/1(LiquidTank1)
  EB2/1 -> Control/5(EmergencyButton)
  MasterTankControl/1(AllowTheTankFilling) -> Logical Operator/2
  Logical Operator/1 -> TankModel/1(LiquidIn)
  LL1/1 -> Memory1/1

== system c00003M_harness/M031/Tank1 ==
  CT1 : Inport
  F1 : Inport  Port=2
  E1 : Inport  Port=3
  MR1 : Inport  Port=4
  T1 : Inport  Port=5
  EB1 : Inport  Port=6
  LL2 : Inport  Port=7
  Control : Subsystem
  Logical Operator : Logic  AllPortsSameDT=off  OutDataTypeStr=boolean
  MasterTankControl : Subsystem
  Memory : Memory
  Memory1 : Memory
  TankModel : Subsystem
  LL1 : Outport
  wires:
  TankModel/1(LiquidLevel) -> Memory/1, LL1/1
  Control/1(LiquidIn) -> Logical Operator/1
  Control/2(LiquidOut) -> TankModel/2(LiquidOut)
  Memory/1 -> Control/7(LiquidLevel), MasterTankControl/1(LiquidTank1)
  MR1/1 -> Control/3(ManualReference)
  CT1/1 -> Control/2(StartMaintenance), Control/1(ControlType)
  F1/1 -> Control/4(Fill)
  E1/1 -> Control/5(Empty)
  Memory1/1 -> MasterTankControl/2(LiquidTank2)
  EB1/1 -> Control/6(EmergencyButton)
  MasterTankControl/1(AllowTheTankFilling) -> Logical Operator/2
  Logical Operator/1 -> TankModel/1(LiquidIn)
  LL2/1 -> Memory1/1
